simulink model "ej10"  (R2023a)
settings: Solver=VariableStepAuto  StartTime=0.0  StopTime=40  RelTol=1e-3
libraries: simulink x2
settings Model: Creator=santi  LastModifiedBy=santi

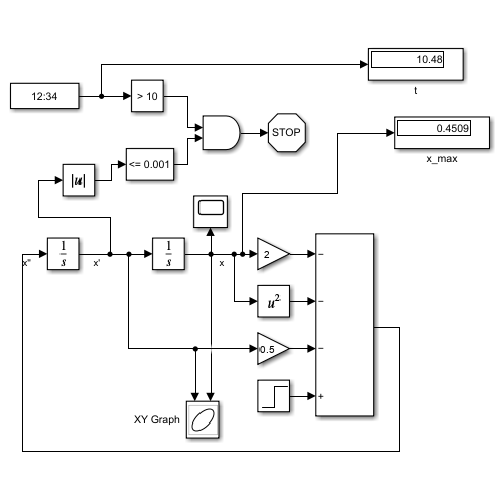
[thumbnail: Simulink's stored preview of the top-level diagram]
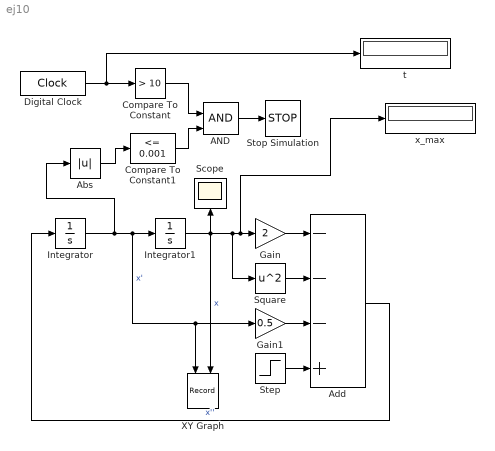
== system ej10 ==
  AND : Logic  IconShape=distinctive  AllPortsSameDT=off  OutDataTypeStr=boolean
  Abs : Abs  SaturateOnIntegerOverflow=off
  Add : Sum  Inputs=---+
  Compare To Constant : simulink/Logic and Bit Operations/Compare To Constant  relop=>  const=10  OutDataTypeStr=boolean
  Compare To Constant1 : simulink/Logic and Bit Operations/Compare To Constant  relop=<=  const=0.001  OutDataTypeStr=boolean
  Digital Clock : DigitalClock  SampleTime=0.001
  Gain : Gain  Gain=2
  Gain1 : Gain  Gain=0.5
  Integrator : Integrator
  Integrator1 : Integrator
  Scope : Scope
  Square : Math  Operator=square
  Step : Step  SampleTime=0
  Stop Simulation : Stop
  XY Graph : Record  VariableName=recordout_XY  RecordToWorkspace=on  FileSettingsInternal="{\"entries\":[{\"content\":{\"excelSettings\":{\"content\":{},\"type\":\"Streamout.ExcelSettings\"}},\"type\":\"Streamout.FileSettingStorage\",\"uuid\":\"\"}],\"packageUris\":[\"http:\\/\\/schema.mathworks.com\\/mf0\\/streamout_blocks\\/R2020a\"],\"version\":\"1.0\"}"  Layout=[1 1]  SignalsInternal="{\"entries\":[{\"content\":{\"signals\":[{\"content\":{\"blockPath\":[],\"dimensions\":[1],\"domain\":\"\",\"lineColor\":\"#a2142f\",\"plots\":[1],\"port\":1,\"sid\":[\"\"],\"signalID\":778,\"signalName\":\"x'\"},\"type\":\"RecordBlkView.Signal\",\"uuid\":\"\"},{\"content\":{\"blockPath\":[],\"dimensions\":[1],\"domain\":\"\",\"lineColor\":\"#139fff\",\"plots\":[1],\"port\":2,\"sid\":[\"\"],\"signalID\":782,\"signalName\":\"x\"},\"type\":\"RecordBlkView.Signal\",\"uuid\":\"\"}]},\"type\":\"RecordBlkView.InputSignals\",\"uuid\":\"\"}],\"packageUris\":[\"http:\\/\\/schema.mathworks.com\\/mf0\\/streamout_blocks\\/R2020a\"],\"version\":\"1.0\"}"  VisualizationBindings="{\"xyplotplugin\":{\"info\":[{\"series\":[{\"bindingParametersList\":[{\"parameter\":\"X-Axis\",\"signalID\":778,\"signalName\":\"x'\"},{\"parameter\":\"Y-Axis\",\"signalID\":782,\"signalName\":\"x\"}],\"seriesID\":9384}],\"subplotID\":1}]}}"  CompatibilityTag=XY
  t : Display
  x_max : Display
  wires:
  Integrator/1 -> Integrator1/1, XY Graph/1, Gain1/1, Abs/1  "x'"
  Integrator1/1 -> XY Graph/2, Scope/1, x_max/1, Gain/1, Square/1  "x"
  Add/1 -> Integrator/1  "x''"
  Step/1 -> Add/4
  Gain1/1 -> Add/3
  Square/1 -> Add/2
  Gain/1 -> Add/1
  Compare To Constant1/1 -> AND/2
  Digital Clock/1 -> t/1, Compare To Constant/1
  Compare To Constant/1 -> AND/1
  Abs/1 -> Compare To Constant1/1
  AND/1 -> Stop Simulation/1
